simulink model "AdaptiveCruiseControl"  (R2020a)
settings: Solver=FixedStepDiscrete  StartTime=0.0  StopTime=100  FixedStep=0.01  RelTol=1e-3  EnableMultiTasking=on
InitFcn:
  | Acceleration_Mode = 0
settings Model: DataDictionary=AdaptiveCruiseControl.sldd  EnableAccessToBaseWorkspace=off  Creator=91968  LastModifiedBy=91968
settings DataIOCC: ReturnWorkspaceOutputs=off
settings OptimizationCC: DefaultParameterBehavior=Inlined  OptimizeBlockIOStorage=off  BufferReuse=off  GlobalBufferReuse=off  ExpressionFolding=off  LocalBlockOutputs=off  LifeSpan=1  EfficientTunableParamExpr=on
settings DebuggingCC: UnderspecifiedInitializationDetection=Classic  MergeDetectMultiDrivingBlocksExec=none  SFUnexpectedBacktrackingDiag=warning  SFNoUnconditionalDefaultTransitionDiag=warning  ArithmeticOperatorsInVariantConditions=warning
settings SFSimCC: SimUseLocalCustomCode=off  MATLABDynamicMemAlloc=off  CustomCodeUndefinedFunction=UseInterfaceOnly
settings RTWCC: SystemTargetFile=ert.tlc  TemplateMakefile=ert_default_tmf  GenerateReport=on  RTWUseLocalCustomCode=off  IncludeHyperlinkInReport=on  LaunchReport=on  GenerateTraceInfo=on  GenerateTraceReport=on  GenerateTraceReportSl=on  GenerateTraceReportSf=on  GenerateTraceReportEml=on
settings CodeAppCC: ForceParamTrailComments=on  IgnoreCustomStorageClasses=off  OperatorAnnotations=on  SimulinkDataObjDesc=on  SFDataObjDesc=on  MATLABFcnDesc=on  InsertBlockDesc=on  StateflowObjectComments=on  MATLABSourceComments=on
settings ERTTargetCC: MultiwordLength=2048  GenerateSampleERTMain=on  InlinedParameterPlacement=NonHierarchical  ERTCustomFileTemplate=example_file_process.tlc
settings ConfigComp: CovMetricSettings=dw  CovHtmlReporting=on  CovSaveCumulativeToWorkspaceVar=on  CovSaveSingleToWorkspaceVar=on  CovExternalEMLEnable=off

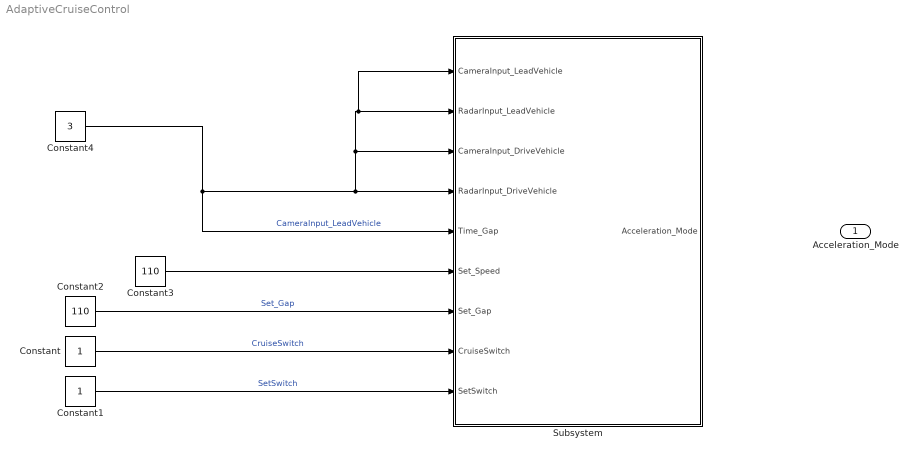
== system AdaptiveCruiseControl ==
  Constant : Constant  OutDataTypeStr=boolean
  Constant1 : Constant  OutDataTypeStr=boolean
  Constant2 : Constant  Value=110  OutDataTypeStr=uint8
  Constant3 : Constant  Value=110  OutDataTypeStr=uint8
  Constant4 : Constant  Value=3  OutDataTypeStr=uint8
  Subsystem : Subsystem
  Acceleration_Mode : Outport  OutMin=0  OutMax=255  OutDataTypeStr=uint8
  wires:
  Constant4/1 -> Subsystem/5(Time_Gap), Subsystem/1("CameraInput_LeadVehicle "), Subsystem/2(RadarInput_LeadVehicle), Subsystem/3(CameraInput_DriveVehicle), Subsystem/4(RadarInput_DriveVehicle)  "CameraInput_LeadVehicle"
  Constant/1 -> Subsystem/8(CruiseSwitch)  "CruiseSwitch"
  Constant1/1 -> Subsystem/9(SetSwitch)  "SetSwitch"
  Constant2/1 -> Subsystem/7(Set_Gap)  "Set_Gap"
  Constant3/1 -> Subsystem/6(Set_Speed)

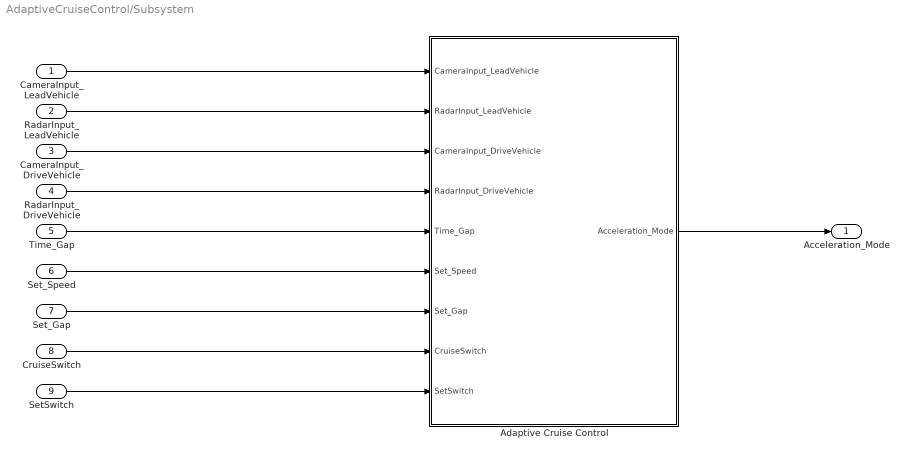
== system AdaptiveCruiseControl/Subsystem ==
  "CameraInput_LeadVehicle " : Inport
  RadarInput_LeadVehicle : Inport  Port=2
  CameraInput_DriveVehicle : Inport  Port=3
  RadarInput_DriveVehicle : Inport  Port=4
  Time_Gap : Inport  Port=5
  Set_Speed : Inport  Port=6
  Set_Gap : Inport  Port=7
  CruiseSwitch : Inport  Port=8
  SetSwitch : Inport  Port=9
  Adaptive Cruise Control : Subsystem
  Acceleration_Mode : Outport
  wires:
  Set_Speed/1 -> Adaptive Cruise Control/6(Set_Speed)
  SetSwitch/1 -> Adaptive Cruise Control/9(SetSwitch)
  "CameraInput_LeadVehicle "/1 -> Adaptive Cruise Control/1("CameraInput_LeadVehicle ")
  Adaptive Cruise Control/1(Acceleration_Mode) -> Acceleration_Mode/1
  Set_Gap/1 -> Adaptive Cruise Control/7(Set_Gap)
  CruiseSwitch/1 -> Adaptive Cruise Control/8(CruiseSwitch)
  Time_Gap/1 -> Adaptive Cruise Control/5(Time_Gap)
  CameraInput_DriveVehicle/1 -> Adaptive Cruise Control/3(CameraInput_DriveVehicle)
  RadarInput_LeadVehicle/1 -> Adaptive Cruise Control/2(RadarInput_LeadVehicle)
  RadarInput_DriveVehicle/1 -> Adaptive Cruise Control/4(RadarInput_DriveVehicle)

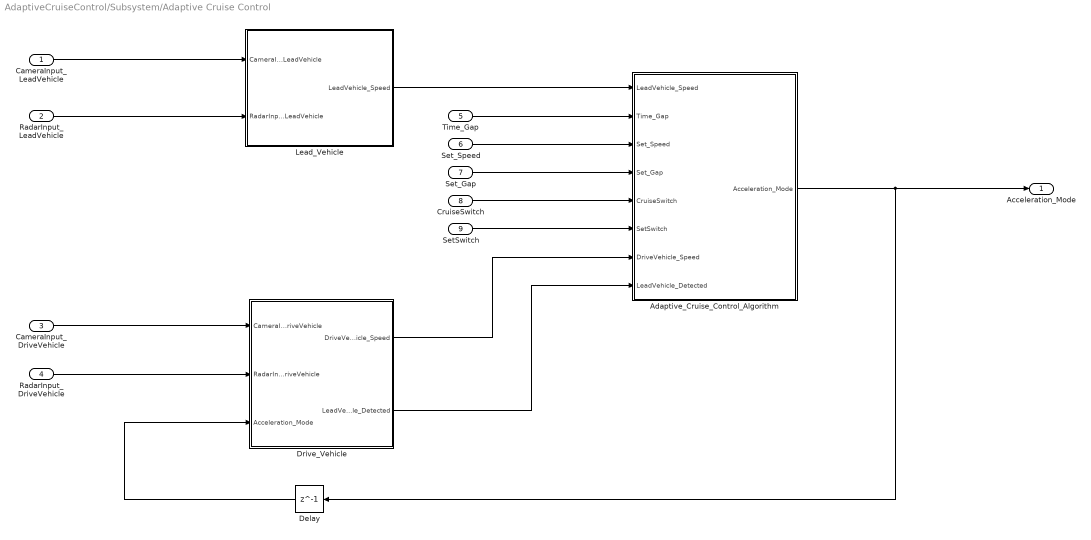
== system AdaptiveCruiseControl/Subsystem/Adaptive Cruise Control ==
  "CameraInput_LeadVehicle " : Inport  OutMin=0  OutMax=255  OutDataTypeStr=uint8
  RadarInput_LeadVehicle : Inport  Port=2  OutMin=0  OutMax=255  OutDataTypeStr=uint8
  CameraInput_DriveVehicle : Inport  Port=3  OutMin=0  OutMax=255  OutDataTypeStr=uint8
  RadarInput_DriveVehicle : Inport  Port=4  OutMin=0  OutMax=255  OutDataTypeStr=uint8
  Time_Gap : Inport  Port=5  OutMin=0  OutMax=255  OutDataTypeStr=uint8
  Set_Speed : Inport  Port=6  OutMin=0  OutMax=255  OutDataTypeStr=uint8
  Set_Gap : Inport  Port=7  OutMin=0  OutMax=255  OutDataTypeStr=uint8
  CruiseSwitch : Inport  Port=8  OutMin=0  OutMax=1  OutDataTypeStr=boolean
  SetSwitch : Inport  Port=9  OutMin=0  OutMax=1  OutDataTypeStr=boolean
  Adaptive_Cruise_Control_Algorithm : Subsystem
  Delay : Delay  DelayLength=1  InitialCondition=0
  Drive_Vehicle : Subsystem
  Lead_Vehicle : Subsystem
  Acceleration_Mode : Outport  OutMin=0  OutMax=255  OutDataTypeStr=uint8
  wires:
  SetSwitch/1 -> Adaptive_Cruise_Control_Algorithm/6(SetSwitch)
  RadarInput_DriveVehicle/1 -> Drive_Vehicle/2(RadarInput_DriveVehicle)
  CameraInput_DriveVehicle/1 -> Drive_Vehicle/1(CameraInput_DriveVehicle)
  Drive_Vehicle/2(LeadVehicle_Detected) -> Adaptive_Cruise_Control_Algorithm/8(LeadVehicle_Detected)
  Drive_Vehicle/1(DriveVehicle_Speed) -> Adaptive_Cruise_Control_Algorithm/7(DriveVehicle_Speed)
  Adaptive_Cruise_Control_Algorithm/1(Acceleration_Mode) -> Acceleration_Mode/1, Delay/1
  Time_Gap/1 -> Adaptive_Cruise_Control_Algorithm/2(Time_Gap)
  RadarInput_LeadVehicle/1 -> Lead_Vehicle/2(RadarInput_LeadVehicle)
  "CameraInput_LeadVehicle "/1 -> Lead_Vehicle/1(CameraInput_LeadVehicle)
  Lead_Vehicle/1(LeadVehicle_Speed) -> Adaptive_Cruise_Control_Algorithm/1(LeadVehicle_Speed)
  Delay/1 -> Drive_Vehicle/3(Acceleration_Mode)
  Set_Speed/1 -> Adaptive_Cruise_Control_Algorithm/3(Set_Speed)
  CruiseSwitch/1 -> Adaptive_Cruise_Control_Algorithm/5(CruiseSwitch)
  Set_Gap/1 -> Adaptive_Cruise_Control_Algorithm/4(Set_Gap)

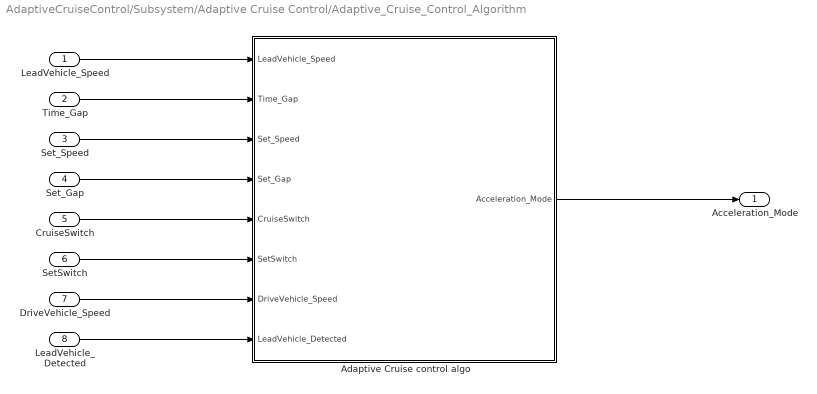
== system AdaptiveCruiseControl/Subsystem/Adaptive Cruise Control/Adaptive_Cruise_Control_Algorithm ==
  LeadVehicle_Speed : Inport  OutMin=0  OutMax=255  OutDataTypeStr=uint8
  Time_Gap : Inport  Port=2
  Set_Speed : Inport  Port=3
  Set_Gap : Inport  Port=4
  CruiseSwitch : Inport  Port=5
  SetSwitch : Inport  Port=6
  DriveVehicle_Speed : Inport  Port=7  OutMin=0  OutMax=255  OutDataTypeStr=uint8
  LeadVehicle_Detected : Inport  Port=8  OutMin=0  OutMax=255  OutDataTypeStr=uint8
  Adaptive Cruise control algo : Stateflow chart  RequirementInfo="{}  %GIDa_5530e465_25c7_4716_b4e3_d6461df02260"  TreatAsAtomicUnit=on
  Acceleration_Mode : Outport  OutMin=0  OutMax=255  OutDataTypeStr=uint8
  wires:
  LeadVehicle_Speed/1 -> Adaptive Cruise control algo/1(LeadVehicle_Speed)
  Set_Gap/1 -> Adaptive Cruise control algo/4(Set_Gap)
  Set_Speed/1 -> Adaptive Cruise control algo/3(Set_Speed)
  Time_Gap/1 -> Adaptive Cruise control algo/2(Time_Gap)
  LeadVehicle_Detected/1 -> Adaptive Cruise control algo/8(LeadVehicle_Detected)
  DriveVehicle_Speed/1 -> Adaptive Cruise control algo/7(DriveVehicle_Speed)
  SetSwitch/1 -> Adaptive Cruise control algo/6(SetSwitch)
  CruiseSwitch/1 -> Adaptive Cruise control algo/5(CruiseSwitch)
  Adaptive Cruise control algo/1(Acceleration_Mode) -> Acceleration_Mode/1

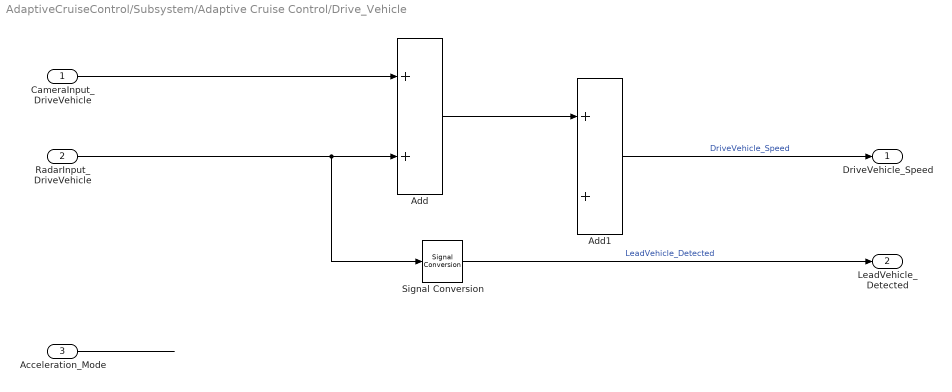
== system AdaptiveCruiseControl/Subsystem/Adaptive Cruise Control/Drive_Vehicle ==
  CameraInput_DriveVehicle : Inport
  RadarInput_DriveVehicle : Inport  Port=2
  Acceleration_Mode : Inport  Port=3
  Add : Sum
  Add1 : Sum
  Signal Conversion : SignalConversion  OverrideOpt=off
  DriveVehicle_Speed : Outport
  LeadVehicle_Detected : Outport  Port=2
  wires:
  RadarInput_DriveVehicle/1 -> Add/2, Signal Conversion/1
  Add/1 -> Add1/1
  Signal Conversion/1 -> LeadVehicle_Detected/1  "LeadVehicle_Detected"
  Add1/1 -> DriveVehicle_Speed/1  "DriveVehicle_Speed"
  CameraInput_DriveVehicle/1 -> Add/1
  Acceleration_Mode/1 -> ?

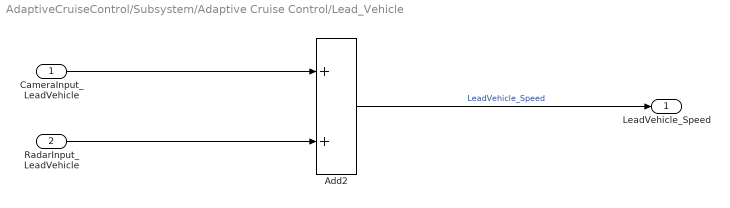
== system AdaptiveCruiseControl/Subsystem/Adaptive Cruise Control/Lead_Vehicle ==
  CameraInput_LeadVehicle : Inport
  RadarInput_LeadVehicle : Inport  Port=2
  Add2 : Sum
  LeadVehicle_Speed : Outport
  wires:
  RadarInput_LeadVehicle/1 -> Add2/2
  CameraInput_LeadVehicle/1 -> Add2/1
  Add2/1 -> LeadVehicle_Speed/1  "LeadVehicle_Speed"

== stateflow chart AdaptiveCruiseControl/Subsystem/Adaptive Cruise Control/Adaptive_Cruise_Control_Algorithm/Adaptive Cruise control algo ==
  state ACC_STANDBY_MODE
    entry:
    Acceleration_Mode = uint8(1);
  state ACC_OFF_MODE
    entry:
    Acceleration_Mode = uint8(0);
  state ACC_ON_MODE
    state LeadVehicle_Not_Detected_Resume
      entry:
      Acceleration_Mode= uint8(1);
    state LeadVehicle_Detected_Resume
      entry:
      Acceleration_Mode= uint8(3);
    state LeadVehicle_Detected_Follow
      entry:
      Acceleration_Mode= uint8(2);
    state LeadVehicle_Not_Detected
      entry:
      Acceleration_Mode= uint8(1);
    state LeadVehicle_Speed_equal_Set_Speed
      entry:
      Acceleration_Mode= uint8(4);
    state LeadVehicle_Speed_lessthan_Set_Speed
      entry:
      Acceleration_Mode= uint8(5);
    (default) -> LeadVehicle_Detected_Follow
    LeadVehicle_Detected_Resume -> LeadVehicle_Not_Detected_Resume [order 1] : [LeadVehicle_Detected ==0]
    LeadVehicle_Detected_Follow -> LeadVehicle_Detected_Resume [order 3] : [(DriveVehicle_Speed==Set_Speed) ...
        | && (LeadVehicle_Speed >= Set_Speed)...
        |  && (Time_Gap>=Set_Gap)]
    LeadVehicle_Speed_lessthan_Set_Speed -> LeadVehicle_Not_Detected_Resume [order 2] : [(LeadVehicle_Detected==0) ...
        | || (DriveVehicle_Speed <= Set_Speed)]
    LeadVehicle_Detected_Resume -> LeadVehicle_Speed_lessthan_Set_Speed [order 2] : [(DriveVehicle_Speed< Set_Speed) ...
        | && (LeadVehicle_Speed > DriveVehicle_Speed)...
        | || (Time_Gap >= Set_Gap)]
    LeadVehicle_Speed_lessthan_Set_Speed -> LeadVehicle_Detected_Resume [order 1] : [(DriveVehicle_Speed< Set_Speed) ...
        | && (LeadVehicle_Speed > DriveVehicle_Speed)...
        | && (Time_Gap >= Set_Gap)]
    LeadVehicle_Detected_Follow -> LeadVehicle_Not_Detected [order 2] : [LeadVehicle_Detected ==0]
    LeadVehicle_Not_Detected -> LeadVehicle_Detected_Follow [order 1] : [(LeadVehicle_Detected==1) && ...
        | (DriveVehicle_Speed == Set_Speed) && ...
        |  (LeadVehicle_Speed >= Set_Speed) &&...
        |  (Time_Gap>=Set_Gap)]
    LeadVehicle_Detected_Follow -> LeadVehicle_Speed_equal_Set_Speed [order 1] : [(LeadVehicle_Detected==1) ...
        | && (LeadVehicle_Speed < Set_Speed)...
        |  || (Time_Gap<Set_Gap)]
    LeadVehicle_Speed_equal_Set_Speed -> LeadVehicle_Not_Detected [order 1] : [(LeadVehicle_Detected==0) && ...
        | (DriveVehicle_Speed == Set_Speed)]
    LeadVehicle_Not_Detected -> LeadVehicle_Speed_equal_Set_Speed [order 2] : [(LeadVehicle_Detected==1) ...
        | && (LeadVehicle_Speed < Set_Speed)...
        |  || (Time_Gap<Set_Gap)]
    LeadVehicle_Speed_lessthan_Set_Speed -> LeadVehicle_Speed_equal_Set_Speed [order 3] : [(LeadVehicle_Speed< Set_Speed) ...
        | && (LeadVehicle_Speed < DriveVehicle_Speed)...
        | || (Time_Gap == 0.75*Set_Gap)]
    LeadVehicle_Speed_equal_Set_Speed -> LeadVehicle_Speed_lessthan_Set_Speed [order 2] : [(LeadVehicle_Speed*1.25 >= DriveVehicle_Speed) ...
        | && (LeadVehicle_Speed*0.75 <= DriveVehicle_Speed)...
        | && (DriveVehicle_Speed < Set_Speed) && (Time_Gap <=1.25*Set_Gap)...
        | && (Time_Gap >= 0.75*Set_Gap)]
  (default) -> ACC_OFF_MODE
  ACC_OFF_MODE -> ACC_STANDBY_MODE : [CruiseSwitch == 1]
  ACC_STANDBY_MODE -> ACC_OFF_MODE [order 1] : [CruiseSwitch==0]
  ACC_ON_MODE -> ACC_STANDBY_MODE : [SetSwitch ==0]
  ACC_STANDBY_MODE -> ACC_ON_MODE [order 2] : [SetSwitch ==1]
  data: LeadVehicle_Speed input uint8; Time_Gap input uint8; Set_Speed input uint8; Set_Gap input uint8; CruiseSwitch input boolean [0..1]; SetSwitch input boolean [0..1]; DriveVehicle_Speed input uint8; LeadVehicle_Detected input uint8; Acceleration_Mode output uint8
